simulink model "Mathmatical_Equation_Time_Domain"  (R2023a)
settings: Solver=VariableStepAuto  StartTime=0.0  StopTime=10.0  RelTol=1e-3
values from neighbouring files (symbols this model uses):
  B = 10    [Mathmatical_Equation_Script.m]
  K = 20    [Mathmatical_Equation_Script.m]
  M = 1    [Mathmatical_Equation_Script.m]
settings Model: Creator=ass1728  LastModifiedBy=ass1728

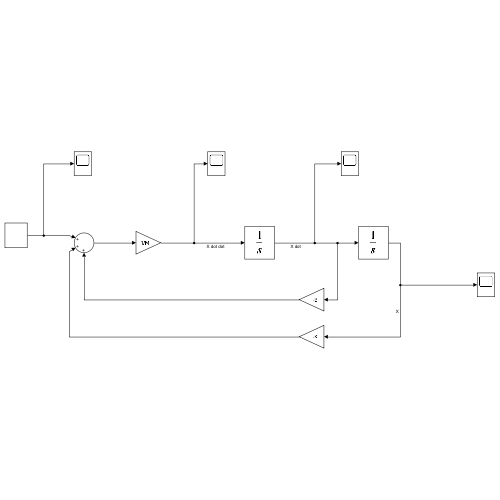
[thumbnail: Simulink's stored preview of the top-level diagram]
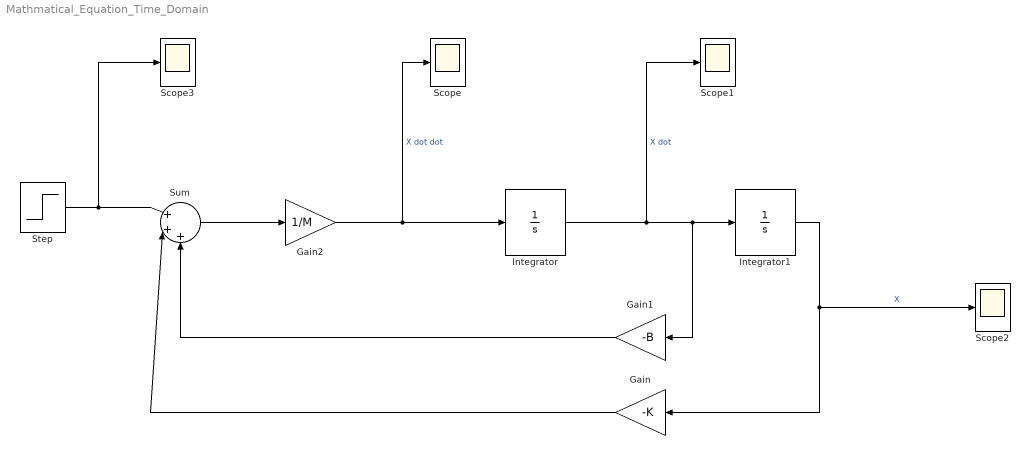
== system Mathmatical_Equation_Time_Domain ==
  Gain : Gain  Gain=-K
  Gain1 : Gain  Gain=-B
  Gain2 : Gain  Gain=1/M
  Integrator : Integrator
  Integrator1 : Integrator
  Scope{,1..3} (4 alike) : Scope
  Step : Step  SampleTime=0
  Sum : Sum  Inputs=|+++
  wires:
  Integrator/1 -> Scope1/1, Gain1/1, Integrator1/1  "X dot"
  Integrator1/1 -> Gain/1, Scope2/1  "X"
  Gain1/1 -> Sum/3
  Gain/1 -> Sum/2
  Sum/1 -> Gain2/1
  Gain2/1 -> Scope/1, Integrator/1  "X dot dot"
  Step/1 -> Scope3/1, Sum/1
